simulink subsystem "station2a"  (R2024b)
settings: Solver=VariableStepAuto  StartTime=0.0  StopTime=10.0  RelTol=1e-3
undefined symbols (not defined in the file): DiscIntNeverNeededParam, h, R3, ResistanceM, Rt4, Ts, Zm
libraries: ee_lib x105, nesl_utility x83, fl_lib x73, simulink x6, simetran x1, powerlib_extras x1
(part 4 of 4)

== system station2a/Subsystem/commfault/Subsystem2/Subsystem1 ==
  in : Inport
  ind : Inport  Port=2
  Constant3 : Constant  Value=[1 0]
  Data Type Conversion : DataTypeConversion  OutDataTypeStr=double  SaturateOnIntegerOverflow=off  RndMeth=Floor
  Relational Operator : RelationalOperator  Operator===  OutDataTypeStr=boolean  InputSameDT=off
  Selector1 : Selector  IndexMode=Zero-based  InputPortWidth=2  IndexOptions=Index vector (port)  Indices=1  OutputSizes=1
  Out1 : Outport
  wires:
  in/1 -> Relational Operator/1
  ind/1 -> Relational Operator/2
  Selector1/1 -> Out1/1
  Constant3/1 -> Selector1/1
  Relational Operator/1 -> Data Type Conversion/1
  Data Type Conversion/1 -> Selector1/2

== system station2a/Subsystem/commfault/Subsystem2/Subsystem10 ==
  in : Inport
  ind : Inport  Port=2
  Constant3 : Constant  Value=[1 0]
  Data Type Conversion : DataTypeConversion  OutDataTypeStr=double  SaturateOnIntegerOverflow=off  RndMeth=Floor
  Relational Operator : RelationalOperator  Operator===  OutDataTypeStr=boolean  InputSameDT=off
  Selector1 : Selector  IndexMode=Zero-based  InputPortWidth=2  IndexOptions=Index vector (port)  Indices=1  OutputSizes=1
  Out1 : Outport
  wires:
  in/1 -> Relational Operator/1
  ind/1 -> Relational Operator/2
  Selector1/1 -> Out1/1
  Constant3/1 -> Selector1/1
  Relational Operator/1 -> Data Type Conversion/1
  Data Type Conversion/1 -> Selector1/2

== system station2a/Subsystem/commfault/Subsystem2/Subsystem11 ==
  in : Inport
  ind : Inport  Port=2
  Constant3 : Constant  Value=[1 0]
  Data Type Conversion : DataTypeConversion  OutDataTypeStr=double  SaturateOnIntegerOverflow=off  RndMeth=Floor
  Relational Operator : RelationalOperator  Operator===  OutDataTypeStr=boolean  InputSameDT=off
  Selector1 : Selector  IndexMode=Zero-based  InputPortWidth=2  IndexOptions=Index vector (port)  Indices=1  OutputSizes=1
  Out1 : Outport
  wires:
  Data Type Conversion/1 -> Selector1/2
  Relational Operator/1 -> Data Type Conversion/1
  Constant3/1 -> Selector1/1
  Selector1/1 -> Out1/1
  ind/1 -> Relational Operator/2
  in/1 -> Relational Operator/1

== system station2a/Subsystem/commfault/Subsystem2/Subsystem2 ==
  in : Inport
  ind : Inport  Port=2
  Constant3 : Constant  Value=[1 0]
  Data Type Conversion : DataTypeConversion  OutDataTypeStr=double  SaturateOnIntegerOverflow=off  RndMeth=Floor
  Relational Operator : RelationalOperator  Operator===  OutDataTypeStr=boolean  InputSameDT=off
  Selector1 : Selector  IndexMode=Zero-based  InputPortWidth=2  IndexOptions=Index vector (port)  Indices=1  OutputSizes=1
  Out1 : Outport
  wires:
  Data Type Conversion/1 -> Selector1/2
  Relational Operator/1 -> Data Type Conversion/1
  Constant3/1 -> Selector1/1
  Selector1/1 -> Out1/1
  ind/1 -> Relational Operator/2
  in/1 -> Relational Operator/1

== system station2a/Subsystem/commfault/Subsystem2/Subsystem3 ==
  in : Inport
  ind : Inport  Port=2
  Constant3 : Constant  Value=[1 0]
  Data Type Conversion : DataTypeConversion  OutDataTypeStr=double  SaturateOnIntegerOverflow=off  RndMeth=Floor
  Relational Operator : RelationalOperator  Operator===  OutDataTypeStr=boolean  InputSameDT=off
  Selector1 : Selector  IndexMode=Zero-based  InputPortWidth=2  IndexOptions=Index vector (port)  Indices=1  OutputSizes=1
  Out1 : Outport
  wires:
  in/1 -> Relational Operator/1
  ind/1 -> Relational Operator/2
  Selector1/1 -> Out1/1
  Constant3/1 -> Selector1/1
  Relational Operator/1 -> Data Type Conversion/1
  Data Type Conversion/1 -> Selector1/2

== system station2a/Subsystem/commfault/Subsystem2/Subsystem4 ==
  in : Inport
  ind : Inport  Port=2
  Constant3 : Constant  Value=[1 0]
  Data Type Conversion : DataTypeConversion  OutDataTypeStr=double  SaturateOnIntegerOverflow=off  RndMeth=Floor
  Relational Operator : RelationalOperator  Operator===  OutDataTypeStr=boolean  InputSameDT=off
  Selector1 : Selector  IndexMode=Zero-based  InputPortWidth=2  IndexOptions=Index vector (port)  Indices=1  OutputSizes=1
  Out1 : Outport
  wires:
  Data Type Conversion/1 -> Selector1/2
  Relational Operator/1 -> Data Type Conversion/1
  Constant3/1 -> Selector1/1
  Selector1/1 -> Out1/1
  ind/1 -> Relational Operator/2
  in/1 -> Relational Operator/1

== system station2a/Subsystem/commfault/Subsystem2/Subsystem5 ==
  in : Inport
  ind : Inport  Port=2
  Constant3 : Constant  Value=[1 0]
  Data Type Conversion : DataTypeConversion  OutDataTypeStr=double  SaturateOnIntegerOverflow=off  RndMeth=Floor
  Relational Operator : RelationalOperator  Operator===  OutDataTypeStr=boolean  InputSameDT=off
  Selector1 : Selector  IndexMode=Zero-based  InputPortWidth=2  IndexOptions=Index vector (port)  Indices=1  OutputSizes=1
  Out1 : Outport
  wires:
  in/1 -> Relational Operator/1
  ind/1 -> Relational Operator/2
  Selector1/1 -> Out1/1
  Constant3/1 -> Selector1/1
  Relational Operator/1 -> Data Type Conversion/1
  Data Type Conversion/1 -> Selector1/2

== system station2a/Subsystem/commfault/Subsystem2/Subsystem6 ==
  in : Inport
  ind : Inport  Port=2
  Constant3 : Constant  Value=[1 0]
  Data Type Conversion : DataTypeConversion  OutDataTypeStr=double  SaturateOnIntegerOverflow=off  RndMeth=Floor
  Relational Operator : RelationalOperator  Operator===  OutDataTypeStr=boolean  InputSameDT=off
  Selector1 : Selector  IndexMode=Zero-based  InputPortWidth=2  IndexOptions=Index vector (port)  Indices=1  OutputSizes=1
  Out1 : Outport
  wires:
  Data Type Conversion/1 -> Selector1/2
  Relational Operator/1 -> Data Type Conversion/1
  Constant3/1 -> Selector1/1
  Selector1/1 -> Out1/1
  ind/1 -> Relational Operator/2
  in/1 -> Relational Operator/1

== system station2a/Subsystem/commfault/Subsystem2/Subsystem7 ==
  in : Inport
  ind : Inport  Port=2
  Constant3 : Constant  Value=[1 0]
  Data Type Conversion : DataTypeConversion  OutDataTypeStr=double  SaturateOnIntegerOverflow=off  RndMeth=Floor
  Relational Operator : RelationalOperator  Operator===  OutDataTypeStr=boolean  InputSameDT=off
  Selector1 : Selector  IndexMode=Zero-based  InputPortWidth=2  IndexOptions=Index vector (port)  Indices=1  OutputSizes=1
  Out1 : Outport
  wires:
  in/1 -> Relational Operator/1
  ind/1 -> Relational Operator/2
  Selector1/1 -> Out1/1
  Constant3/1 -> Selector1/1
  Relational Operator/1 -> Data Type Conversion/1
  Data Type Conversion/1 -> Selector1/2

== system station2a/Subsystem/commfault/Subsystem2/Subsystem8 ==
  in : Inport
  ind : Inport  Port=2
  Constant3 : Constant  Value=[1 0]
  Data Type Conversion : DataTypeConversion  OutDataTypeStr=double  SaturateOnIntegerOverflow=off  RndMeth=Floor
  Relational Operator : RelationalOperator  Operator===  OutDataTypeStr=boolean  InputSameDT=off
  Selector1 : Selector  IndexMode=Zero-based  InputPortWidth=2  IndexOptions=Index vector (port)  Indices=1  OutputSizes=1
  Out1 : Outport
  wires:
  Data Type Conversion/1 -> Selector1/2
  Relational Operator/1 -> Data Type Conversion/1
  Constant3/1 -> Selector1/1
  Selector1/1 -> Out1/1
  ind/1 -> Relational Operator/2
  in/1 -> Relational Operator/1

== system station2a/Subsystem/commfault/Subsystem2/Subsystem9 ==
  in : Inport
  ind : Inport  Port=2
  Constant3 : Constant  Value=[1 0]
  Data Type Conversion : DataTypeConversion  OutDataTypeStr=double  SaturateOnIntegerOverflow=off  RndMeth=Floor
  Relational Operator : RelationalOperator  Operator===  OutDataTypeStr=boolean  InputSameDT=off
  Selector1 : Selector  IndexMode=Zero-based  InputPortWidth=2  IndexOptions=Index vector (port)  Indices=1  OutputSizes=1
  Out1 : Outport
  wires:
  Data Type Conversion/1 -> Selector1/2
  Relational Operator/1 -> Data Type Conversion/1
  Constant3/1 -> Selector1/1
  Selector1/1 -> Out1/1
  ind/1 -> Relational Operator/2
  in/1 -> Relational Operator/1
